simulink model "crazyflie"  (R2017b)
settings: Solver=FixedStepDiscrete  StartTime=0.0  StopTime=10  FixedStep=T  RelTol=1e-3
values from neighbouring files (symbols this model uses):
  g = 9.82    [setup_lqr.m]
undefined symbols (not defined in the file or in its folder): Kc, Q, R_acc, R_LPS, sensor_position, T
libraries: simulink_extras x3
settings Model: PauseTimes=7  Creator=Zrean  LastModifiedBy=viktor
settings OptimizationCC: DefaultParameterBehavior=Inlined  UseDivisionForNetSlopeComputation=on  UseFloatMulNetSlope=on  UseSpecifiedMinMax=on  InlineInvariantSignals=on  PassReuseOutputArgsAs=Individual arguments  ZeroExternalMemoryAtStartup=off  ZeroInternalMemoryAtStartup=off  NoFixptDivByZeroProtection=on  EfficientFloat2IntCast=on  LifeSpan=1
settings DebuggingCC: AlgebraicLoopMsg=error  ParameterTunabilityLossMsg=error
settings HardwareCC: ProdBitPerPointer=32  ProdBitPerSizeT=32  ProdBitPerPtrDiffT=32  ProdLargestAtomicInteger=Long  ProdLargestAtomicFloat=Double  ProdWordSize=32  ProdHWDeviceType=ARM Compatible->ARM Cortex
settings ModelReferenceCC: ModelReferenceNumInstancesAllowed=Single
settings SFSimCC: MATLABDynamicMemAlloc=off
settings RTWCC: SystemTargetFile=ert.tlc  GenCodeOnly=on  TemplateMakefile=ert_default_tmf  GenerateReport=on  BuildConfiguration=Faster Runs  IncludeHyperlinkInReport=on  LaunchReport=on  GenerateTraceInfo=on  GenerateTraceReport=on  GenerateTraceReportSl=on  GenerateTraceReportSf=on  GenerateTraceReportEml=on  GenerateCodeMetricsReport=on
settings CodeAppCC: ForceParamTrailComments=on  IgnoreCustomStorageClasses=off  OperatorAnnotations=on  SimulinkDataObjDesc=on  SFDataObjDesc=on  MATLABFcnDesc=on  CustomSymbolStrGlobalVar=rt$N$M  CustomSymbolStrType=$N$M  CustomSymbolStrFcn=$N$M$F  CustomSymbolStrMacro=$N$M  InsertBlockDesc=on  StateflowObjectComments=on  MATLABSourceComments=on
settings ERTTargetCC: TargetLangStandard=C99 (ISO)  CodeReplacementLibrary=ARM trigfcn  MultiwordLength=2048  CombineSignalStateStructs=on  SuppressErrorStatus=on  SupportAbsoluteTime=off  SupportNonFinite=off  SupportComplex=off  InlinedParameterPlacement=NonHierarchical  ERTCustomFileTemplate=crazyflie_wrapper_loco.tlc  ERTFilePackagingFormat=CompactWithDataFile
settings SimscapeCC: SimscapeNormalizeSystem=off

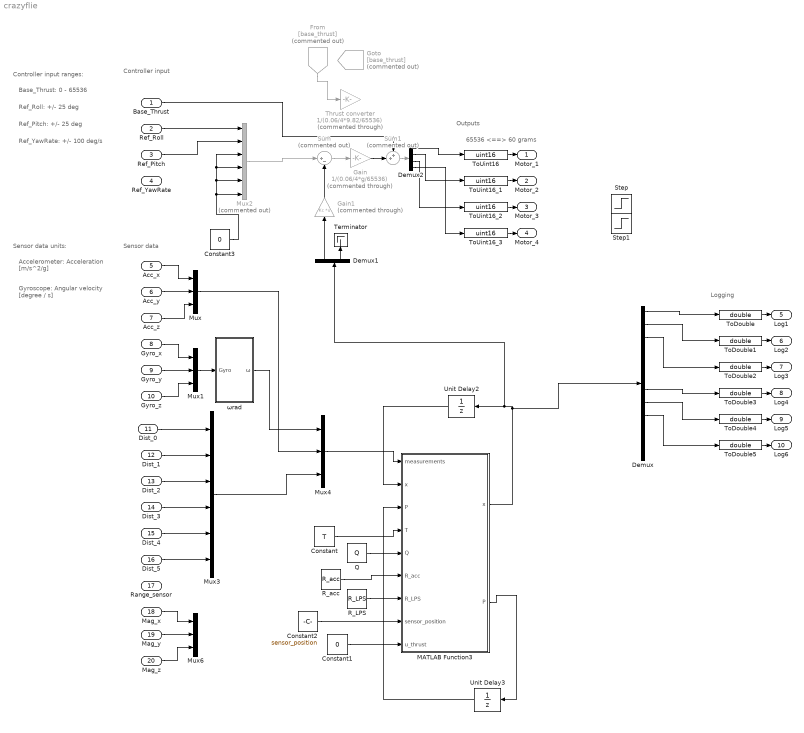
== system crazyflie ==
  note: 65536 <==> 60 grams
  note: Logging
  note: Outputs
  note: Sensor data
  note: Controller input
  note: Ref_Roll: +/- 25 deg
  note: Base_Thrust: 0 - 65536
  note: Ref_Pitch: +/- 25 deg
  note: Ref_YawRate: +/- 100 deg/s
  note: Controller input ranges:
  note: Gyroscope:
      | Angular velocity [degree / s]
  note: Accelerometer:
      | Acceleration [m/s^2/g]
  note: Sensor data units:
  Base_Thrust : Inport  OutDataTypeStr=double
  Ref_Roll : Inport  Port=2  OutDataTypeStr=double
  Ref_Pitch : Inport  Port=3  OutDataTypeStr=double
  Ref_YawRate : Inport  Port=4  OutDataTypeStr=double
  Acc_x : Inport  Port=5  OutDataTypeStr=double  PortDimensions=1
  Acc_y : Inport  Port=6  OutDataTypeStr=double  PortDimensions=1
  Acc_z : Inport  Port=7  OutDataTypeStr=double  PortDimensions=1
  Gyro_x : Inport  Port=8  OutDataTypeStr=double  PortDimensions=1
  Gyro_y : Inport  Port=9  OutDataTypeStr=double  PortDimensions=1
  Gyro_z : Inport  Port=10  OutDataTypeStr=double  PortDimensions=1
  Dist_0 : Inport  Port=11  OutDataTypeStr=double  PortDimensions=1
  Dist_1 : Inport  Port=12  OutDataTypeStr=double  PortDimensions=1
  Dist_2 : Inport  Port=13  OutDataTypeStr=double  PortDimensions=1
  Dist_3 : Inport  Port=14  OutDataTypeStr=double  PortDimensions=1
  Dist_4 : Inport  Port=15  OutDataTypeStr=double  PortDimensions=1
  Dist_5 : Inport  Port=16  OutDataTypeStr=double  PortDimensions=1
  Range_sensor : Inport  Port=17  OutDataTypeStr=double  PortDimensions=1
  Mag_x : Inport  Port=18  OutDataTypeStr=double  PortDimensions=1
  Mag_y : Inport  Port=19  OutDataTypeStr=double  PortDimensions=1
  Mag_z : Inport  Port=20  OutDataTypeStr=double  PortDimensions=1
  "  ωrad " : Subsystem
  Constant : Constant  Value=T
  Constant1 : Constant  Value=0
  Constant2 : Constant  Value=sensor_position
  Constant3 : Constant  Value=0
  Demux : Demux  Outputs=12
  Demux1 : Demux  Outputs=2
  Demux2 : Demux
  From : From  Commented=on  GotoTag=base_thrust
  Gain : Gain  Commented=through  Gain=1/(0.06/4*g/65536)
  Gain1 : Gain  Commented=through  Gain=Kc  Multiplication=Matrix(K*u) (u vector)
  Goto : Goto  Commented=on  GotoTag=base_thrust
  MATLAB Function3 : MATLAB Function  TreatAsAtomicUnit=on
  Mux{,1,4,6} (4 alike) : Mux  Inputs=3
  Mux2 : Mux  Commented=on  Inputs=6
  Mux3 : Mux  Inputs=6
  Q : Constant  Value=Q
  R_LPS : Constant  Value=R_LPS
  R_acc : Constant  Value=R_acc
  Step : Step  Time=2  After=2000  SampleTime=T
  Step1 : Step  After=0  SampleTime=T
  Sum : Sum  Commented=on  Inputs=|+-
  Sum1 : Sum  Commented=on  Inputs=++|
  Terminator : Terminator
  "Thrust converter " : Gain  Commented=through  Gain=1/(0.06/4*9.82/65536)
  ToDouble{,1..5} (6 alike) : DataTypeConversion  OutDataTypeStr=double  SaturateOnIntegerOverflow=on
  ToUint16 : DataTypeConversion  OutDataTypeStr=uint16  SaturateOnIntegerOverflow=on
  ToUint16_1 : DataTypeConversion  OutDataTypeStr=uint16  SaturateOnIntegerOverflow=on
  ToUint16_2 : DataTypeConversion  OutDataTypeStr=uint16  SaturateOnIntegerOverflow=on
  ToUint16_3 : DataTypeConversion  OutDataTypeStr=uint16  SaturateOnIntegerOverflow=on
  Unit Delay2 : UnitDelay  InitialCondition=zeros(12,1)  SampleTime=-1
  Unit Delay3 : UnitDelay  InitialCondition=eye(12)  SampleTime=-1
  Motor_1 : Outport  OutDataTypeStr=uint16  LockScale=on
  Motor_2 : Outport  Port=2  OutDataTypeStr=uint16  LockScale=on
  Motor_3 : Outport  Port=3  OutDataTypeStr=uint16  LockScale=on
  Motor_4 : Outport  Port=4  OutDataTypeStr=uint16  LockScale=on
  Log1 : Outport  Port=5  OutDataTypeStr=double
  Log2 : Outport  Port=6  OutDataTypeStr=double
  Log3 : Outport  Port=7  OutDataTypeStr=double
  Log4 : Outport  Port=8  OutDataTypeStr=double
  Log5 : Outport  Port=9  OutDataTypeStr=double
  Log6 : Outport  Port=10  OutDataTypeStr=double
  wires:
  ToUint16/1 -> Motor_1/1
  ToUint16_1/1 -> Motor_2/1
  ToUint16_2/1 -> Motor_3/1
  ToUint16_3/1 -> Motor_4/1
  ToDouble/1 -> Log1/1
  ToDouble1/1 -> Log2/1
  ToDouble2/1 -> Log3/1
  ToDouble3/1 -> Log4/1
  ToDouble4/1 -> Log5/1
  ToDouble5/1 -> Log6/1
  Acc_y/1 -> Mux/2
  Gyro_z/1 -> Mux1/3
  Acc_z/1 -> Mux/3
  Gyro_x/1 -> Mux1/1
  Gyro_y/1 -> Mux1/2
  Acc_x/1 -> Mux/1
  Ref_Roll/1 -> Mux2/1
  Ref_Pitch/1 -> Mux2/2
  From/1 -> "Thrust converter "/1
  Dist_0/1 -> Mux3/1
  Dist_1/1 -> Mux3/2
  Dist_2/1 -> Mux3/3
  Dist_3/1 -> Mux3/4
  Dist_4/1 -> Mux3/5
  Dist_5/1 -> Mux3/6
  Mux1/1 -> "  ωrad "/1(Gyro)
  Mux3/1 -> Mux4/3
  "  ωrad "/1("  ω") -> Mux4/1
  Mag_x/1 -> Mux6/1
  Mag_y/1 -> Mux6/2
  Mag_z/1 -> Mux6/3
  MATLAB Function3/1(x) -> Demux/1, Demux1/1, Unit Delay2/1
  Mux4/1 -> MATLAB Function3/1(measurements)
  MATLAB Function3/2(P) -> Unit Delay3/1
  Constant/1 -> MATLAB Function3/4(T)
  R_acc/1 -> MATLAB Function3/6(R_acc)
  Q/1 -> MATLAB Function3/5(Q)
  R_LPS/1 -> MATLAB Function3/7(R_LPS)
  Constant1/1 -> MATLAB Function3/9(u_thrust)
  Constant2/1 -> MATLAB Function3/8(sensor_position)
  Unit Delay2/1 -> MATLAB Function3/2("x ")
  Unit Delay3/1 -> MATLAB Function3/3("P ")
  Mux/1 -> Mux4/2
  Demux/1 -> ToDouble/1
  Demux/2 -> ToDouble1/1
  Demux/3 -> ToDouble2/1
  Demux/7 -> ToDouble3/1
  Demux/8 -> ToDouble4/1
  Demux/9 -> ToDouble5/1
  Base_Thrust/1 -> Sum1/1
  Demux2/4 -> ToUint16_3/1
  Sum/1 -> Gain/1
  Demux1/1 -> Gain1/1
  Gain1/1 -> Sum/2
  Gain/1 -> Sum1/2
  Sum1/1 -> Demux2/1
  Demux2/1 -> ToUint16/1
  Demux2/2 -> ToUint16_1/1
  Demux2/3 -> ToUint16_2/1
  Constant3/1 -> Mux2/3, Mux2/4, Mux2/5, Mux2/6
  Mux2/1 -> Sum/1
  Demux1/2 -> Terminator/1

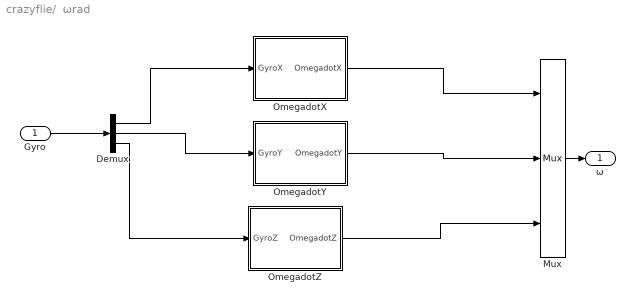
== system crazyflie/  ωrad  ==
  Gyro : Inport
  Demux : Demux  Outputs=3
  Mux : Mux  Inputs=3
  OmegadotX : Subsystem
  OmegadotY : Subsystem
  OmegadotZ : Subsystem
  "  ω" : Outport
  wires:
  OmegadotZ/1("OmegadotZ ") -> Mux/3
  Demux/1 -> OmegadotX/1("GyroX ")
  OmegadotX/1("OmegadotX ") -> Mux/1
  Demux/3 -> OmegadotZ/1("GyroZ ")
  OmegadotY/1("OmegadotY ") -> Mux/2
  Gyro/1 -> Demux/1
  Demux/2 -> OmegadotY/1("GyroY ")
  Mux/1 -> "  ω"/1

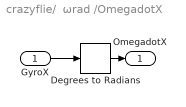
== system crazyflie/  ωrad /OmegadotX ==
  "GyroX " : Inport
  Degrees to Radians : simulink_extras/Transformations/Degrees to Radians
  "OmegadotX " : Outport
  wires:
  Degrees to Radians/1 -> "OmegadotX "/1
  "GyroX "/1 -> Degrees to Radians/1

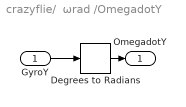
== system crazyflie/  ωrad /OmegadotY ==
  "GyroY " : Inport
  Degrees to Radians : simulink_extras/Transformations/Degrees to Radians
  "OmegadotY " : Outport
  wires:
  Degrees to Radians/1 -> "OmegadotY "/1
  "GyroY "/1 -> Degrees to Radians/1

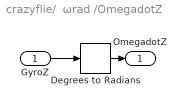
== system crazyflie/  ωrad /OmegadotZ ==
  "GyroZ " : Inport
  Degrees to Radians : simulink_extras/Transformations/Degrees to Radians
  "OmegadotZ " : Outport
  wires:
  Degrees to Radians/1 -> "OmegadotZ "/1
  "GyroZ "/1 -> Degrees to Radians/1

== matlab function crazyflie/MATLAB Function3 ==
  data: measurements input; x output; P output; x input; P input; T input; Q input; R_acc input; R_LPS input; sensor_position input; u_thrust input

function [x, P] = ExtendedKalmanFilter(measurements,x,P,T,Q,R_acc,R_LPS,sensor_position,u_thrust)
%NONLINEARKALMANFILTER Filters measurement sequence Y using a 
% non-linear Kalman filter. 
% TODO Implement Zranger
%Input:
%   Y                       [m x 1] Measurement sequence for times 1,...,N
%   statePrior        [n x 1] Prior mean for time 0
%   priorCovariance    [n x n] Prior covariance
%   motionModel                     Motion model function handle
%
%Output:
%   xf          [n x 1]     Filtered estimates for times 1,...,N
%   Pf          [n x n ] Filter error convariance
%

[x, P]=predictionGyro(x, measurements, P, T,Q); %Prediction With Gyro-

[x, P]=predictionLPS(x, P, T,Q,u_thrust);                                                %Prediction With LPS
[x, P]=updateAcc(x, measurements, P, T,R_acc);                                                 % Update With accelerometer
[x, P]=updateLPS(x, measurements, sensor_position, P, T,R_LPS);                    % Update With LPS


end
